simulink model "ESC251_MATLABTakeHome_Q2BD"  (R2025b)
settings: Solver=VariableStepAuto  StartTime=0.0  StopTime=10  RelTol=1e-3
values from neighbouring files (symbols this model uses):
  b = 4000    [ESC251_HW4.m]    (also in ESC251_TakeHomeQ2.m = b_vals(i); ESC251_TakeHomeQ2d.m = 40000; SystemsFinalProject_linearized.m = 0.5; SystemsFinalProject_linearized_ramp.m = 0.5)
  k = 80.8e5    (= 8080000)    [ESC251_TakeHomeQ2.m]    (also in ESC251_TakeHomeQ2d.m)
  m = 0.033    [ESC251_LabAssign.m]    (also in ESC251_TakeHomeQ1.m; ESC251_TakeHomeQ2.m = 3000; ESC251_TakeHomeQ2d.m = 3000; SystemsFinalProject_linearized.m = 0.4)
  u1 = 0:0.01:1    [ESC251_HW4.m]    (also in ESC251_TakeHomeQ2.m = 20000; ESC251_TakeHomeQ2d.m = 0)
  v0 = 0.0    (= 0)    [ESC251_TakeHomeQ2d.m]
  x0 = [0, 100]    [ESC251_LabAssign.m]    (also in ESC251_TakeHomeQ1.m = [0; 0]; ESC251_TakeHomeQ2d.m = 0.01)
libraries: simulink x1
settings Model: Creator=mydkm  LastModifiedBy=mydkm

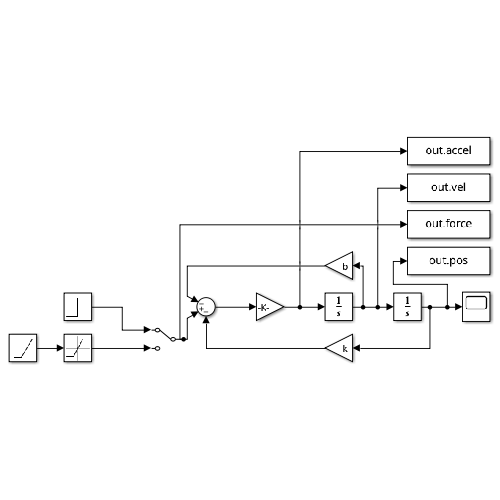
[thumbnail: Simulink's stored preview of the top-level diagram]
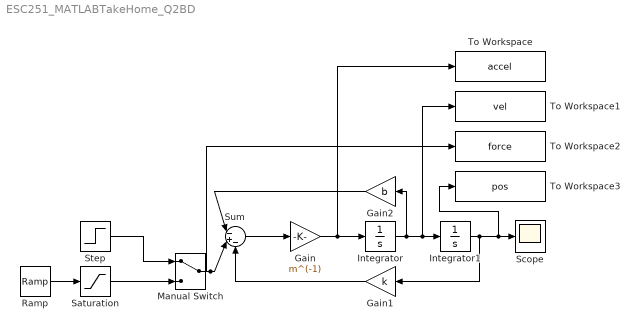
== system ESC251_MATLABTakeHome_Q2BD ==
  Gain : Gain  Gain=m^(-1)
  Gain1 : Gain  Gain=k
  Gain2 : Gain  Gain=b
  Integrator : Integrator  InitialCondition=v0
  Integrator1 : Integrator  InitialCondition=x0
  Manual Switch : ManualSwitch
  Ramp : simulink/Sources/Ramp  slope=20000  start=0  InitialOutput=0
  Saturation : Saturate  UpperLimit=20000  LowerLimit=0
  Scope : Scope
  Step : Step  Time=0  After=u1  SampleTime=0
  Sum : Sum  Inputs=|-+-
  To Workspace : ToWorkspace  VariableName=accel  SaveFormat=Timeseries  SampleTime=-1
  To Workspace1 : ToWorkspace  VariableName=vel  SaveFormat=Timeseries  SampleTime=-1
  To Workspace2 : ToWorkspace  VariableName=force  SaveFormat=Timeseries  SampleTime=-1
  To Workspace3 : ToWorkspace  VariableName=pos  SaveFormat=Timeseries  SampleTime=-1
  wires:
  Sum/1 -> Gain/1
  Gain/1 -> To Workspace/1, Integrator/1
  Integrator/1 -> Gain2/1, To Workspace1/1, Integrator1/1
  Integrator1/1 -> Gain1/1, To Workspace3/1, Scope/1
  Gain1/1 -> Sum/3
  Gain2/1 -> Sum/1
  Step/1 -> Manual Switch/1
  Ramp/1 -> Saturation/1
  Saturation/1 -> Manual Switch/2
  Manual Switch/1 -> Sum/2, To Workspace2/1
